simulink model "drone_controller"  (R2017a)
settings: Solver=FixedStepAuto  StartTime=0.0  StopTime=10.0  FixedStep=0.0001  RelTol=1e-3
libraries: simulink x1
settings Model: Creator=mrais  LastModifiedBy=mrais

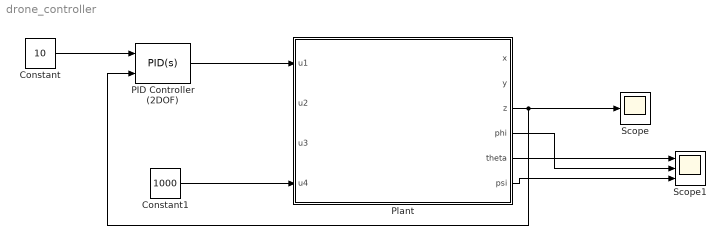
== system drone_controller ==
  Constant : Constant  Value=10
  Constant1 : Constant  Value=1000
  PID Controller (2DOF) : simulink/Continuous/PID Controller (2DOF)  Controller=PID  TimeDomain=Continuous-time  SampleTime=-1  IntegratorMethod=Forward Euler  FilterMethod=Forward Euler  Form=Parallel  UseFilter=on  ControllerParametersSource=internal  P=20  I=0  D=20  N=100  b=1  c=1  InitialConditionSource=internal  InitialConditionForIntegrator=0  InitialConditionForFilter=0  ExternalReset=none  LimitOutput=off  UpperSaturationLimit=inf  LowerSaturationLimit=-inf  LinearizeAsGain=on  AntiWindupMode=none  Kb=1  TrackingMode=off  Kt=1  PParamMin=[]  PParamMax=[]  IParamMin=[]  IParamMax=[]  DParamMin=[]  DParamMax=[]  NParamMin=[]  NParamMax=[]  bParamMin=[]  bParamMax=[]  cParamMin=[]  cParamMax=[]  KbParamMin=[]  KbParamMax=[]  KtParamMin=[]  KtParamMax=[]  POutMin=[]  POutMax=[]  IOutMin=[]  IOutMax=[]  DOutMin=[]  DOutMax=[]  NOutMin=[]  NOutMax=[]  bOutMin=[]  bOutMax=[]  cOutMin=[]  cOutMax=[]  KbOutMin=[]  KbOutMax=[]  KtOutMin=[]  KtOutMax=[]  IntegratorOutMin=[]  IntegratorOutMax=[]  FilterOutMin=[]  FilterOutMax=[]  SumOutMin=[]  SumOutMax=[]  Sum1OutMin=[]  Sum1OutMax=[]  Sum2OutMin=[]  Sum2OutMax=[]  Sum3OutMin=[]  Sum3OutMax=[]  SumI1OutMin=[]  SumI1OutMax=[]  SumI2OutMin=[]  SumI2OutMax=[]  SumI3OutMin=[]  SumI3OutMax=[]  SumDOutMin=[]  SumDOutMax=[]  SaturationOutMin=[]  SaturationOutMax=[]  IntegratorContinuousStateAttributes=''  IntegratorStateMustResolveToSignalObject=off  IntegratorRTWStateStorageClass=Auto  FilterContinuousStateAttributes=''  FilterStateMustResolveToSignalObject=off  FilterRTWStateStorageClass=Auto  DifferentiatorICPrevScaledInput=0  DifferentiatorOutMin=[]  DifferentiatorOutMax=[]  InitialConditionSetting=State (most efficient)
  Plant : Subsystem
  Scope : Scope
  Scope1 : Scope  NumInputPorts=3
  wires:
  Plant/3(z) -> PID Controller (2DOF)/2, Scope/1
  Constant/1 -> PID Controller (2DOF)/1
  Plant/6(psi) -> Scope1/3
  Plant/5(theta) -> Scope1/1
  Plant/4(phi) -> Scope1/2
  Constant1/1 -> Plant/4(u4)
  PID Controller (2DOF)/1 -> Plant/1(u1)

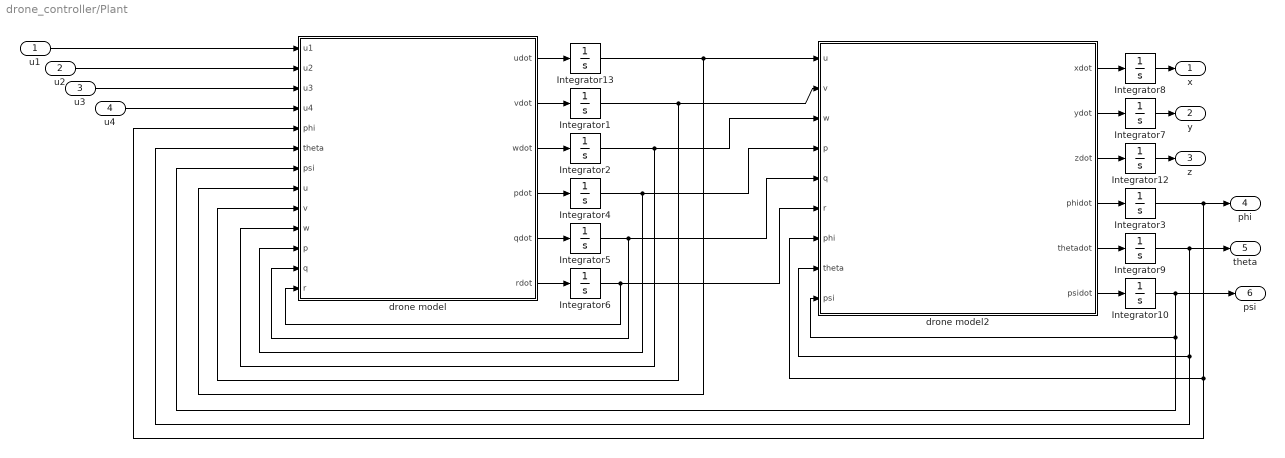
== system drone_controller/Plant ==
  u1 : Inport
  u2 : Inport  Port=2
  u3 : Inport  Port=3
  u4 : Inport  Port=4
  Integrator{1..2,7..8,12..13} (6 alike) : Integrator
  Integrator{3..6,9..10} (6 alike) : Integrator  WrapState=on  WrappedStateUpperValue=2*pi  WrappedStateLowerValue=0
  drone model : MATLAB Function  TreatAsAtomicUnit=on
  drone model2 : MATLAB Function  TreatAsAtomicUnit=on
  x : Outport
  y : Outport  Port=2
  z : Outport  Port=3
  phi : Outport  Port=4
  theta : Outport  Port=5
  psi : Outport  Port=6
  wires:
  drone model/1(udot) -> Integrator13/1
  Integrator9/1 -> theta/1, drone model2/8(theta), drone model/6(theta)
  u1/1 -> drone model/1(u1)
  drone model/6(rdot) -> Integrator6/1
  drone model/4(pdot) -> Integrator4/1
  Integrator3/1 -> phi/1, drone model2/7(phi), drone model/5(phi)
  drone model2/4(phidot) -> Integrator3/1
  drone model2/5(thetadot) -> Integrator9/1
  drone model2/3(zdot) -> Integrator12/1
  Integrator10/1 -> psi/1, drone model2/9(psi), drone model/7(psi)
  u3/1 -> drone model/3(u3)
  Integrator4/1 -> drone model2/4(p), drone model/11(p)
  Integrator5/1 -> drone model2/5(q), drone model/12(q)
  drone model/2(vdot) -> Integrator1/1
  drone model2/1(xdot) -> Integrator8/1
  drone model/3(wdot) -> Integrator2/1
  Integrator13/1 -> drone model/8(u), drone model2/1(u)
  Integrator6/1 -> drone model2/6(r), drone model/13(r)
  Integrator2/1 -> drone model2/3(w), drone model/10(w)
  u4/1 -> drone model/4(u4)
  drone model/5(qdot) -> Integrator5/1
  Integrator1/1 -> drone model2/2(v), drone model/9(v)
  Integrator8/1 -> x/1
  u2/1 -> drone model/2(u2)
  Integrator7/1 -> y/1
  Integrator12/1 -> z/1
  drone model2/2(ydot) -> Integrator7/1
  drone model2/6(psidot) -> Integrator10/1

== matlab function drone_controller/Plant/drone model2 ==
  data: xdot output; ydot output; u input; v input; w input; p input; q input; r input; zdot output; phidot output; thetadot output; psidot output; phi input; theta input; psi input
function [xdot,ydot,zdot,phidot,thetadot,psidot] = BaseSwap(u,v,w,p,q,r,phi,theta,psi)

RT = [cos(psi)*cos(phi) - sin(psi)*cos(theta)*sin(phi)  ,   -cos(psi)*sin(phi) - sin(psi)*cos(theta)*cos(phi)  , sin(psi)*cos(theta), 0, 0, 0;
      sin(psi)*cos(phi) + cos(psi)*cos(theta)*sin(phi)  , -sin(psi)*sin(phi) + cos(psi)*cos(theta)*cos(phi)    , -cos(psi)*sin(theta), 0, 0, 0;
      sin(theta)*sin(phi)                               ,  sin(theta)*cos(phi)                                 ,  cos(theta), 0, 0, 0
      0, 0, 0, 1, sin(phi)*tan(theta), cos(phi)*tan(theta);
      0, 0, 0, 0, cos(phi)           , -sin(phi);
      0, 0, 0, 0, sin(phi)*sec(theta), cos(phi)*sec(theta);
     ];
    
    
X = RT*[u,v,w,p,q,r]';
xdot = X(1);
ydot = X(2);
zdot = X(3);
phidot = X(4);
thetadot = X(5);
psidot = X(6);

end

== matlab function drone_controller/Plant/drone model ==
  data: u1 input; udot output; u2 input; u3 input; u4 input; phi input; theta input; psi input; u input; v input; w input; p input; q input; r input; vdot output; wdot output; pdot output; qdot output; rdot output
function [udot,vdot,wdot, pdot, qdot, rdot]  = model(u1, u2, u3, u4, phi,theta, psi,u, v , w, p, q, r)
g = 9.81; % en m/s²
M = 0.2;  % masse en kg
Ix = 1; Iy = 1; Iz = 0.5; % inertie
Omega = 500; % en rad/s
Jtp = 1; % a voir

udot = (v*r - w*q) + g*sin(theta);
vdot = (w*p - u*r) - g*cos(theta)*sin(phi);
wdot = (u*q - v*p) - g*cos(theta)*cos(phi) + u1/M;
pdot = q*r*(Iy - Iz)/Ix - Jtp*q*Omega/Ix + u2/Ix; 
qdot = p*r*(Iz - Ix)/Iy - Jtp*p*Omega/Iy + u3/Iy; 
rdot = p*q*(Ix - Iy)/Iz + u4/Iz;


end
